simulink model "VCU_board_v8"  (R2019b)
settings: Solver=VariableStepAuto  StartTime=0.0  StopTime=300  RelTol=1e-3
undefined symbols (not defined in the file): canChannel
libraries: canmsglib x46, canlib x40
(part 1 of 2)
settings Model: EnablePacing=on  PacingRate=14  Creator=n10488456  LastModifiedBy=n10228748

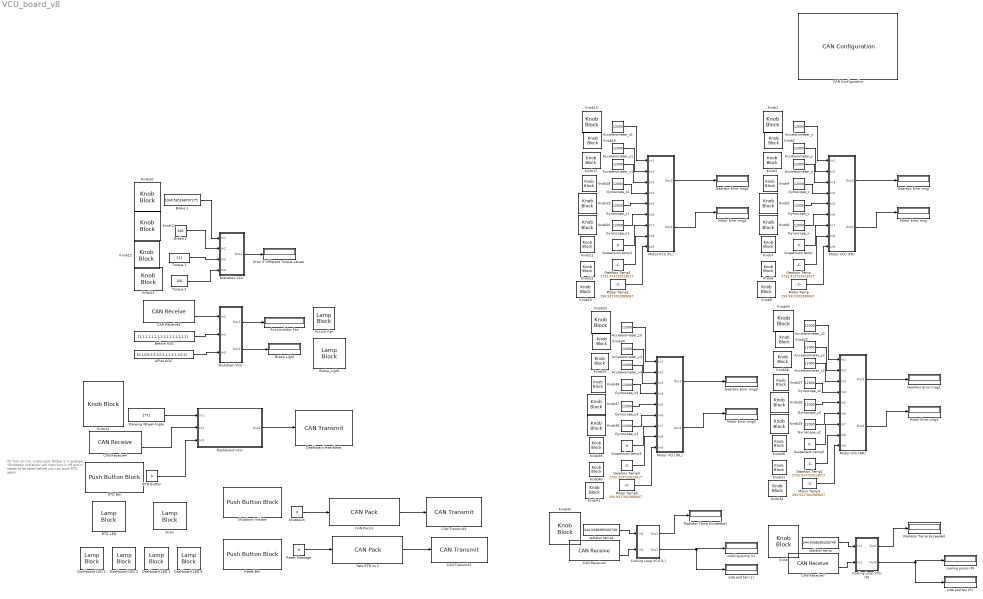
== system VCU_board_v8 ==
  note: To Turn on Car, make sure 'Brake 1' is pushed.
      | 'Shutdown initiation' will then turn it off and it needs to be reset before you can push RTD again.
  AFter ADC : Constant  Value=[0,1,0,0,1,0,1,0,1,1,1,1,1,1,0,1]
  Accelerometer_x{,1..3} (4 alike) : Constant  Value=12000  OutDataTypeStr=uint16
  Accelerometer_y{,1..3} (4 alike) : Constant  Value=12000  OutDataTypeStr=uint16
  Accelerometer_z{,1..3} (4 alike) : Constant  Value=12000  OutDataTypeStr=uint16
  Accum Fan : LampBlock
  Accumulator Fan : Display
  Before ADC : Constant  Value=[1,1,1,1,1,1,1,1,1,1,1,1,1,1,1,1]
  Brake 1 : Constant  Value=1040.565268707275
  Brake 2 : Constant  Value=100
  Brake Light : Display
  Brake_Light : LampBlock
  Brakebox VCU : Subsystem
  CAN Configuration : canlib/CAN Configuration  BlockHandle=69.0009  Device=MathWorks Virtual 1 (Channel 1)  DeviceMenu=MathWorks Virtual 1 (Channel 1)  ObjConstructor=canChannel('MathWorks', 'Virtual 1', 1)  BusSpeed=1000000  EnableBitParameters=off  AckMode=Normal
      settings: SourceProductName=Vehicle Network Toolbox  SourceProductBaseCode=VN
  CAN Pack3 : canmsglib/CAN Pack  MsgList=(none)  MsgName=Shutdown Notif  MsgIDType=Standard (11-bit identifier)  MsgIdentifier=62  MsgLength=1  Remote=off  ApplyMinMax=off  BusOutput=off  SignalInfo={ 'Signal1', '0', '1', 'LE', 'unsigned', 'Standard', '0', '1', '0', '-Inf', 'Inf' }
      settings: SourceProductName=Vehicle Network Toolbox  SourceProductBaseCode=VN  DataFormat=manually specified signals
  CAN Receive1 : canlib/CAN Receive  BlockHandle=71.0007  Device=MathWorks Virtual 1 (Channel 1)  DeviceMenu=MathWorks Virtual 1 (Channel 1)  ObjConstructor=canChannel('MathWorks', 'Virtual 1', 1)  EnableStandardIDsFilter=off  StdIDsCombo=Allow only  StandardIDs=[41 61]  EnableExtendedIDsFilter=off  ExtIDsCombo=Allow all  ExtendedIDs=0  SampleTime=0.01  MsgsPerTimestep=all  InternalFilterUpdateStatus=on  BusOutput=off
      settings: SourceProductName=Vehicle Network Toolbox  SourceProductBaseCode=VN
  CAN Receive4 : canlib/CAN Receive  BlockHandle=72.0004  Device=MathWorks Virtual 1 (Channel 1)  DeviceMenu=MathWorks Virtual 1 (Channel 1)  ObjConstructor=canChannel('MathWorks', 'Virtual 1', 1)  EnableStandardIDsFilter=off  StdIDsCombo=Allow only  StandardIDs=[22 51 61 62]  EnableExtendedIDsFilter=off  ExtIDsCombo=Allow all  ExtendedIDs=0  SampleTime=0.01  MsgsPerTimestep=all  InternalFilterUpdateStatus=on  BusOutput=off
      settings: SourceProductName=Vehicle Network Toolbox  SourceProductBaseCode=VN
  CAN Receive5 : canlib/CAN Receive  BlockHandle=73.0004  Device=MathWorks Virtual 1 (Channel 1)  DeviceMenu=MathWorks Virtual 1 (Channel 1)  ObjConstructor=canChannel('MathWorks', 'Virtual 1', 1)  EnableStandardIDsFilter=off  StdIDsCombo=Allow only  StandardIDs=[41 51 61]  EnableExtendedIDsFilter=off  ExtIDsCombo=Allow all  ExtendedIDs=0  SampleTime=0.01  MsgsPerTimestep=all  InternalFilterUpdateStatus=on  BusOutput=off
      settings: SourceProductName=Vehicle Network Toolbox  SourceProductBaseCode=VN
  CAN Receive7 : canlib/CAN Receive  BlockHandle=74.0004  Device=MathWorks Virtual 1 (Channel 1)  DeviceMenu=MathWorks Virtual 1 (Channel 1)  ObjConstructor=canChannel('MathWorks', 'Virtual 1', 1)  EnableStandardIDsFilter=off  StdIDsCombo=Allow only  StandardIDs=[41 61]  EnableExtendedIDsFilter=off  ExtIDsCombo=Allow all  ExtendedIDs=0  SampleTime=0.01  MsgsPerTimestep=all  InternalFilterUpdateStatus=on  BusOutput=off
      settings: SourceProductName=Vehicle Network Toolbox  SourceProductBaseCode=VN
  CAN Transmit1 : canlib/CAN Transmit  BlockHandle=76.0004  Device=MathWorks Virtual 1 (Channel 1)  DeviceMenu=MathWorks Virtual 1 (Channel 1)  ObjConstructor=canChannel('MathWorks', 'Virtual 1', 1)  EnablePeriodicTransmit=on  MessagePeriod=0.250
      settings: SourceProductName=Vehicle Network Toolbox  SourceProductBaseCode=VN
  CAN Transmit3 : canlib/CAN Transmit  BlockHandle=77.0004  Device=MathWorks Virtual 1 (Channel 1)  DeviceMenu=MathWorks Virtual 1 (Channel 1)  ObjConstructor=canChannel('MathWorks', 'Virtual 1', 1)  EnablePeriodicTransmit=on  MessagePeriod=0.250
      settings: SourceProductName=Vehicle Network Toolbox  SourceProductBaseCode=VN
  Cooling Loop VCU (L) : Subsystem
  Cooling Loop VCU (R) : Subsystem
  Dashboard Heartbeat : canlib/CAN Transmit  BlockHandle=209.0004  Device=MathWorks Virtual 1 (Channel 1)  DeviceMenu=MathWorks Virtual 1 (Channel 1)  ObjConstructor=canChannel('MathWorks', 'Virtual 1', 1)  EnablePeriodicTransmit=on  MessagePeriod=0.250
      settings: SourceProductName=Vehicle Network Toolbox  SourceProductBaseCode=VN
  Dashboard LED {1..4} (4 alike) : LampBlock
  Dashboard VCU : Subsystem
  Error if different Torque values : Display
  Gearbox Error msg{,1..3} (4 alike) : Display
  Gearbox Temp{,1..3} (4 alike) : Constant  Value=2732.414722614017  OutDataTypeStr=uint16
  Gyroscope_x{,1..3} (4 alike) : Constant  Value=12000  OutDataTypeStr=uint16
  Gyroscope_y{,1..3} (4 alike) : Constant  Value=12000  OutDataTypeStr=uint16
  Gyroscope_z{,1..3} (4 alike) : Constant  Value=12000  OutDataTypeStr=uint16
  Knob{,7..14,21..23,30..32,39..42} (19 alike) : KnobBlock  ScaleMax=4095
  Knob{1..6,15..20,24..29,33..38} (24 alike) : KnobBlock  ScaleMax=65535
  Motor Error msg{,1..3} (4 alike) : Display
  Motor Temp{,1..3} (4 alike) : Constant  Value=294.9317002989067  OutDataTypeStr=uint16
  Motor VCU (FL) : Subsystem
  Motor VCU (FR) : Subsystem
  Motor VCU (RL) : Subsystem
  Motor VCU (RR) : Subsystem
  RTD Btn : PushButtonBlock  ButtonText=RTD Button
  RTD Button : Constant  Value=0  OutDataTypeStr=boolean  SampleTime=0.1
  RTD LED : LampBlock
  Radiator Temp Exceeded : Display
  Radiator Temp Exceeded1 : Display
  Reset Btn : PushButtonBlock  ButtonText=Reset Button
  Reset Message : Constant  Value=0
  Sets RTD to 2 : canmsglib/CAN Pack  MsgList=(none)  MsgName=RTD Notif  MsgIDType=Standard (11-bit identifier)  MsgIdentifier=61  MsgLength=1  Remote=off  ApplyMinMax=off  BusOutput=off  SignalInfo={ 'Signal1', '0', '1', 'LE', 'unsigned', 'Standard', '0', '1', '0', '-Inf', 'Inf' }
      settings: SourceProductName=Vehicle Network Toolbox  SourceProductBaseCode=VN  DataFormat=manually specified signals
  Shutdown : Constant  Value=0
  Shutdown Initiate : PushButtonBlock  ButtonText=Shutdown Initiate
  Shutdown VCU : Subsystem
  Siren : LampBlock
  Stereing Wheel Angle : Constant  Value=1771  OutDataTypeStr=uint16  SampleTime=0.1
  Suspension temp{,1..3} (4 alike) : Constant  Value=0  OutDataTypeStr=uint16
  Torque 1 : Constant  Value=111
  Torque 2 : Constant  Value=100
  cooling pump (L) : Display
  cooling pump (R) : Display
  radiator temp : Constant  Value=244.5438395200749  OutDataTypeStr=uint16
  radiator temp1 : Constant  Value=244.5438395200749  OutDataTypeStr=uint16
  side pod fan (L) : Display
  side pod fan (R) : Display
  wires:
  Accelerometer_z/1 -> Motor VCU (FR)/1(In1)
  Accelerometer_y/1 -> Motor VCU (FR)/2(In2)
  Accelerometer_x/1 -> Motor VCU (FR)/3(In3)
  Gyroscope_z/1 -> Motor VCU (FR)/4(In4)
  Gyroscope_y/1 -> Motor VCU (FR)/5(In5)
  Gyroscope_x/1 -> Motor VCU (FR)/6(In6)
  Suspension temp/1 -> Motor VCU (FR)/7(In7)
  Gearbox Temp/1 -> Motor VCU (FR)/8(In8)
  Motor Temp/1 -> Motor VCU (FR)/9(In9)
  Motor VCU (FR)/1(Out3) -> Gearbox Error msg/1
  Motor VCU (FR)/2(Out4) -> Motor Error msg/1
  Brakebox VCU/1(Out2) -> Error if different Torque values/1
  Brake 2/1 -> Brakebox VCU/2(In2)
  Brake 1/1 -> Brakebox VCU/1(In1)
  Torque 2/1 -> Brakebox VCU/4(In4)
  Torque 1/1 -> Brakebox VCU/3(In3)
  CAN Receive4/2 -> Dashboard VCU/2(In2)
  Stereing Wheel Angle/1 -> Dashboard VCU/1(In1)
  Dashboard VCU/1(Out1) -> Dashboard Heartbeat/1
  RTD Button/1 -> Dashboard VCU/3(In3)
  Cooling Loop VCU (R)/2(Out3) -> side pod fan (R)/1, cooling pump (R)/1
  radiator temp/1 -> Cooling Loop VCU (R)/1(In1)
  CAN Receive7/2 -> Cooling Loop VCU (R)/2(In2)
  Cooling Loop VCU (R)/1(Out1) -> Radiator Temp Exceeded/1
  CAN Receive5/2 -> Shutdown VCU/1(In2)
  Shutdown VCU/2(Out2) -> Brake Light/1
  AFter ADC/1 -> Shutdown VCU/3(In5)
  Shutdown VCU/1(Out1) -> Accumulator Fan/1
  Before ADC/1 -> Shutdown VCU/2(In3)
  Shutdown/1 -> CAN Pack3/1
  CAN Pack3/1 -> CAN Transmit3/1
  Reset Message/1 -> Sets RTD to 2/1
  Sets RTD to 2/1 -> CAN Transmit1/1
  Accelerometer_y1/1 -> Motor VCU (FL)/2(In2)
  Motor Temp1/1 -> Motor VCU (FL)/9(In9)
  Gearbox Temp1/1 -> Motor VCU (FL)/8(In8)
  Gyroscope_z1/1 -> Motor VCU (FL)/4(In4)
  Motor VCU (FL)/1(Out3) -> Gearbox Error msg1/1
  Suspension temp1/1 -> Motor VCU (FL)/7(In7)
  Accelerometer_z1/1 -> Motor VCU (FL)/1(In1)
  Accelerometer_x1/1 -> Motor VCU (FL)/3(In3)
  Motor VCU (FL)/2(Out4) -> Motor Error msg1/1
  Gyroscope_x1/1 -> Motor VCU (FL)/6(In6)
  Gyroscope_y1/1 -> Motor VCU (FL)/5(In5)
  Accelerometer_y2/1 -> Motor VCU (RR)/2(In2)
  Motor Temp2/1 -> Motor VCU (RR)/9(In9)
  Gearbox Temp2/1 -> Motor VCU (RR)/8(In8)
  Gyroscope_z2/1 -> Motor VCU (RR)/4(In4)
  Motor VCU (RR)/1(Out3) -> Gearbox Error msg2/1
  Suspension temp2/1 -> Motor VCU (RR)/7(In7)
  Accelerometer_z2/1 -> Motor VCU (RR)/1(In1)
  Accelerometer_x2/1 -> Motor VCU (RR)/3(In3)
  Motor VCU (RR)/2(Out4) -> Motor Error msg2/1
  Gyroscope_x2/1 -> Motor VCU (RR)/6(In6)
  Gyroscope_y2/1 -> Motor VCU (RR)/5(In5)
  Accelerometer_y3/1 -> Motor VCU (RL)/2(In2)
  Motor Temp3/1 -> Motor VCU (RL)/9(In9)
  Gearbox Temp3/1 -> Motor VCU (RL)/8(In8)
  Gyroscope_z3/1 -> Motor VCU (RL)/4(In4)
  Motor VCU (RL)/1(Out3) -> Gearbox Error msg3/1
  Suspension temp3/1 -> Motor VCU (RL)/7(In7)
  Accelerometer_z3/1 -> Motor VCU (RL)/1(In1)
  Accelerometer_x3/1 -> Motor VCU (RL)/3(In3)
  Motor VCU (RL)/2(Out4) -> Motor Error msg3/1
  Gyroscope_x3/1 -> Motor VCU (RL)/6(In6)
  Gyroscope_y3/1 -> Motor VCU (RL)/5(In5)
  Cooling Loop VCU (L)/1(Out1) -> Radiator Temp Exceeded1/1
  radiator temp1/1 -> Cooling Loop VCU (L)/1(In1)
  Cooling Loop VCU (L)/2(Out3) -> side pod fan (L)/1, cooling pump (L)/1
  CAN Receive1/2 -> Cooling Loop VCU (L)/2(In2)

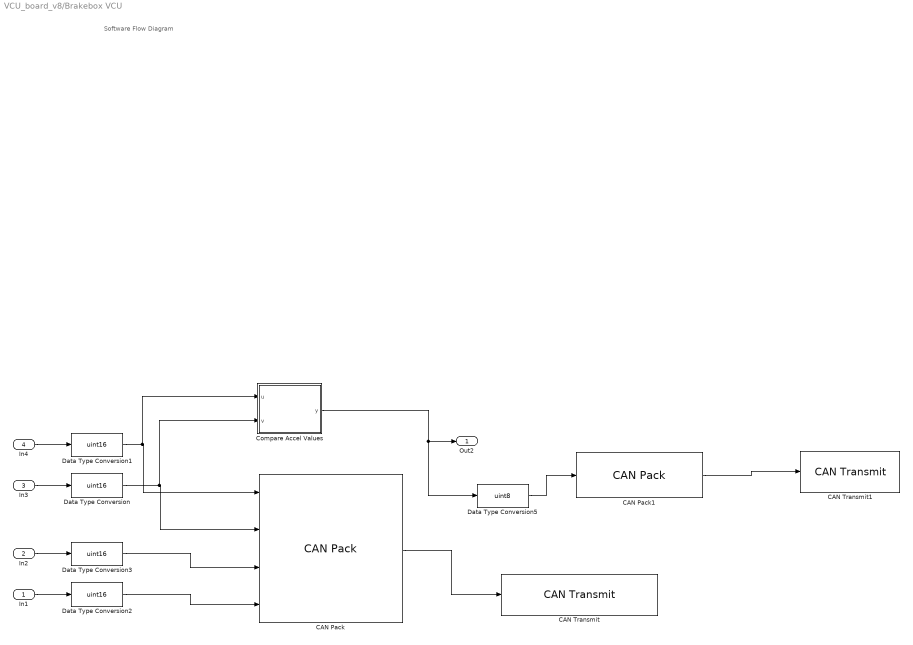
== system VCU_board_v8/Brakebox VCU ==
  note: Software Flow Diagram
  In1 : Inport
  In2 : Inport  Port=2
  In3 : Inport  Port=3
  In4 : Inport  Port=4
  CAN Pack : canmsglib/CAN Pack  MsgList=(none)  MsgName=CAN Msg  MsgIDType=Standard (11-bit identifier)  MsgIdentifier=51  MsgLength=6  Remote=off  ApplyMinMax=off  BusOutput=off  SignalInfo={ 'Torque2', '0', '12', 'LE', 'unsigned', 'Standard', '0', '1', '0', '-Inf', 'Inf'; 'Torque1', '12', '12', 'LE', 'unsigned', 'Standard', '0', '1', '0', '-Inf', 'Inf'; 'BrakePos', '24', '12', 'LE', 'unsigned', 'Standard', '0', '1', '0', '-Inf', 'Inf'; 'BrakePres', '36', '12', 'LE', 'unsigned', 'Standard', '0', '1', '0', '-Inf', 'Inf' }
      settings: SourceProductName=Vehicle Network Toolbox  SourceProductBaseCode=VN  DataFormat=manually specified signals
  CAN Pack1 : canmsglib/CAN Pack  MsgList=(none)  MsgName=CAN Msg  MsgIDType=Standard (11-bit identifier)  MsgIdentifier=52  MsgLength=8  Remote=off  ApplyMinMax=off  BusOutput=off  SignalInfo="{  }"
      settings: SourceProductName=Vehicle Network Toolbox  SourceProductBaseCode=VN  DataFormat=raw data
  CAN Transmit : canlib/CAN Transmit  BlockHandle=19.0002  Device=MathWorks Virtual 1 (Channel 1)  DeviceMenu=MathWorks Virtual 1 (Channel 1)  ObjConstructor=canChannel('MathWorks', 'Virtual 1', 1)  EnablePeriodicTransmit=on  MessagePeriod=0.250
      settings: SourceProductName=Vehicle Network Toolbox  SourceProductBaseCode=VN
  CAN Transmit1 : canlib/CAN Transmit  BlockHandle=20.0002  Device=MathWorks Virtual 1 (Channel 1)  DeviceMenu=MathWorks Virtual 1 (Channel 1)  ObjConstructor=canChannel('MathWorks', 'Virtual 1', 1)  EnablePeriodicTransmit=on  MessagePeriod=0.250
      settings: SourceProductName=Vehicle Network Toolbox  SourceProductBaseCode=VN
  Compare Accel Values : MATLAB Function  TreatAsAtomicUnit=on
  Data Type Conversion{,1..3} (4 alike) : DataTypeConversion  OutDataTypeStr=uint16
  Data Type Conversion5 : DataTypeConversion  OutDataTypeStr=uint8
  Out2 : Outport
  wires:
  In2/1 -> Data Type Conversion3/1
  Data Type Conversion/1 -> Compare Accel Values/2(v), CAN Pack/2
  Data Type Conversion1/1 -> Compare Accel Values/1(u), CAN Pack/1
  In3/1 -> Data Type Conversion/1
  In1/1 -> Data Type Conversion2/1
  Compare Accel Values/1(y) -> Data Type Conversion5/1, Out2/1
  In4/1 -> Data Type Conversion1/1
  CAN Pack/1 -> CAN Transmit/1
  CAN Pack1/1 -> CAN Transmit1/1
  Data Type Conversion5/1 -> CAN Pack1/1
  Data Type Conversion2/1 -> CAN Pack/4
  Data Type Conversion3/1 -> CAN Pack/3

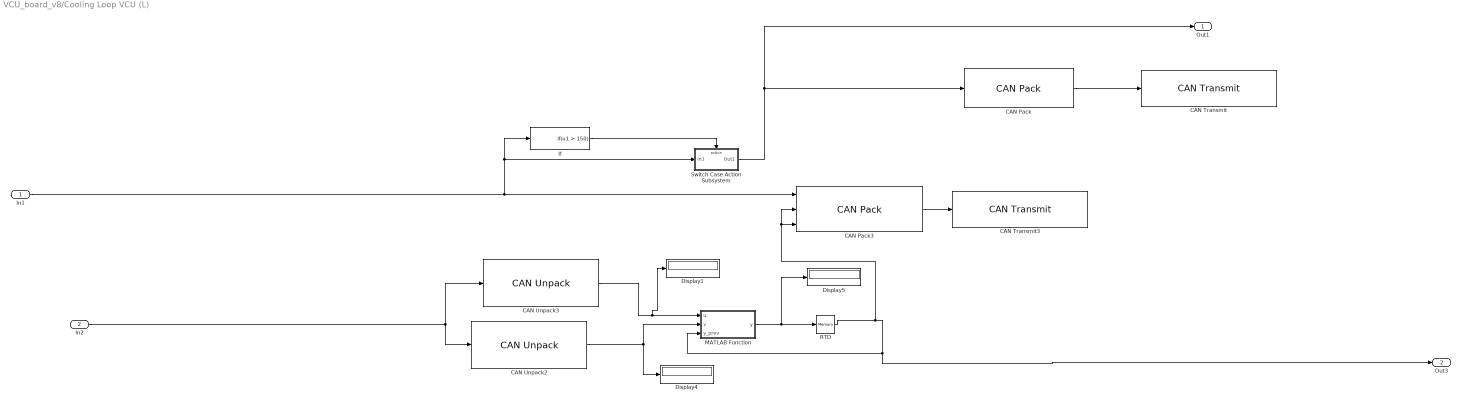
== system VCU_board_v8/Cooling Loop VCU (L) ==
  In1 : Inport
  In2 : Inport  Port=2
  CAN Pack : canmsglib/CAN Pack  MsgList=(none)  MsgName=Error RadiatorT L  MsgIDType=Standard (11-bit identifier)  MsgIdentifier=322  MsgLength=1  Remote=off  ApplyMinMax=off  BusOutput=off  SignalInfo={ 'Signal1', '0', '1', 'LE', 'unsigned', 'Standard', '0', '1', '0', '-Inf', 'Inf' }
      settings: SourceProductName=Vehicle Network Toolbox  SourceProductBaseCode=VN  DataFormat=manually specified signals
  CAN Pack3 : canmsglib/CAN Pack  MsgList=(none)  MsgName=Cooling Loop Heartbeat L  MsgIDType=Standard (11-bit identifier)  MsgIdentifier=312  MsgLength=2  Remote=off  ApplyMinMax=off  BusOutput=off  SignalInfo={ 'RadiatorT', '0', '12', 'LE', 'unsigned', 'Standard', '0', '1', '0', '-Inf', 'Inf'; 'SideFan', '12', '1', 'LE', 'unsigned', 'Standard', '0', '1', '0', '-Inf', 'Inf'; 'Pump', '13', '1', 'LE', 'unsigned', 'Standard', '0', '1', '0', '-Inf', 'Inf' }
      settings: SourceProductName=Vehicle Network Toolbox  SourceProductBaseCode=VN  DataFormat=manually specified signals
  CAN Transmit : canlib/CAN Transmit  BlockHandle=78.0002  Device=MathWorks Virtual 1 (Channel 1)  DeviceMenu=MathWorks Virtual 1 (Channel 1)  ObjConstructor=canChannel('MathWorks', 'Virtual 1', 1)  EnablePeriodicTransmit=on  MessagePeriod=0.250
      settings: SourceProductName=Vehicle Network Toolbox  SourceProductBaseCode=VN
  CAN Transmit3 : canlib/CAN Transmit  BlockHandle=79.0002  Device=MathWorks Virtual 1 (Channel 1)  DeviceMenu=MathWorks Virtual 1 (Channel 1)  ObjConstructor=canChannel('MathWorks', 'Virtual 1', 1)  EnablePeriodicTransmit=on  MessagePeriod=0.250
      settings: SourceProductName=Vehicle Network Toolbox  SourceProductBaseCode=VN
  CAN Unpack2 : canmsglib/CAN Unpack  MsgList=(none)  MsgName=Reset Notif  MsgIDType=Standard (11-bit identifier)  MsgIdentifier=61  MsgLength=1  SignalInfo={ 'Reset', '0', '1', 'LE', 'unsigned', 'Standard', '0', '1', '0', '-Inf', 'Inf' }  IDPort=off  TimestampPort=off  ErrorPort=off  RemotePort=off  LengthPort=off  StatusPort=off  ApplyMinMax=off
      settings: SourceProductName=Vehicle Network Toolbox  SourceProductBaseCode=VN
  CAN Unpack3 : canmsglib/CAN Unpack  MsgList=(none)  MsgName=RTD Notif  MsgIDType=Standard (11-bit identifier)  MsgIdentifier=41  MsgLength=3  SignalInfo={ 'RTD', '0', '1', 'LE', 'unsigned', 'Standard', '0', '1', '0', '-Inf', 'Inf' }  IDPort=off  TimestampPort=off  ErrorPort=off  RemotePort=off  LengthPort=off  StatusPort=off  ApplyMinMax=off
      settings: SourceProductName=Vehicle Network Toolbox  SourceProductBaseCode=VN
  Display1 : Display
  Display4 : Display
  Display5 : Display
  If : If  IfExpression=u1 > 150  ShowElse=off
  MATLAB Function : MATLAB Function  TreatAsAtomicUnit=on
  RTD : Memory  InheritSampleTime=on
  Switch Case Action Subsystem : Subsystem  TreatAsAtomicUnit=on
  Out1 : Outport
  Out3 : Outport  Port=2
  wires:
  In1/1 -> CAN Pack3/1, If/1, Switch Case Action Subsystem/1(In1)
  Switch Case Action Subsystem/1(Out1) -> CAN Pack/1, Out1/1
  CAN Pack/1 -> CAN Transmit/1
  CAN Pack3/1 -> CAN Transmit3/1
  If/1 -> Switch Case Action Subsystem/Action
  CAN Unpack2/1 -> Display4/1, MATLAB Function/2(v)
  CAN Unpack3/1 -> Display1/1, MATLAB Function/1(u)
  In2/1 -> CAN Unpack3/1, CAN Unpack2/1
  MATLAB Function/1(y) -> Display5/1, RTD/1
  RTD/1 -> Out3/1, MATLAB Function/3(y_prev), CAN Pack3/3, CAN Pack3/2

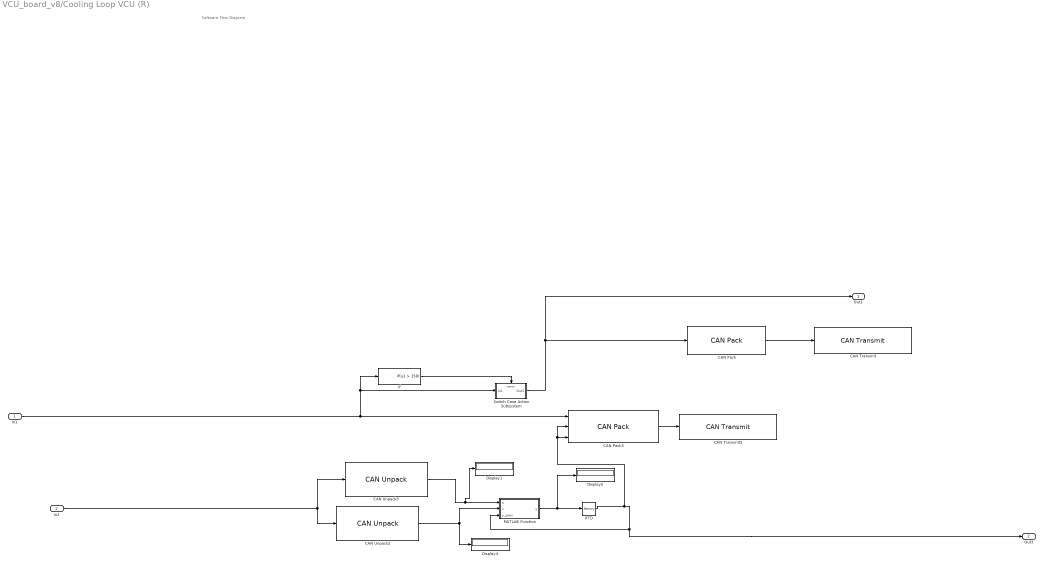
== system VCU_board_v8/Cooling Loop VCU (R) ==
  note: Software Flow Diagram
  In1 : Inport
  In2 : Inport  Port=2
  CAN Pack : canmsglib/CAN Pack  MsgList=(none)  MsgName=Error RadiatorT  MsgIDType=Standard (11-bit identifier)  MsgIdentifier=321  MsgLength=1  Remote=off  ApplyMinMax=off  BusOutput=off  SignalInfo={ 'Signal1', '0', '1', 'LE', 'unsigned', 'Standard', '0', '1', '0', '-Inf', 'Inf' }
      settings: SourceProductName=Vehicle Network Toolbox  SourceProductBaseCode=VN  DataFormat=manually specified signals
  CAN Pack3 : canmsglib/CAN Pack  MsgList=(none)  MsgName=Cooling Loop Heartbeat  MsgIDType=Standard (11-bit identifier)  MsgIdentifier=311  MsgLength=2  Remote=off  ApplyMinMax=off  BusOutput=off  SignalInfo={ 'RadiatorT', '0', '12', 'LE', 'unsigned', 'Standard', '0', '1', '0', '-Inf', 'Inf'; 'SideFan', '12', '1', 'LE', 'unsigned', 'Standard', '0', '1', '0', '-Inf', 'Inf'; 'Pump', '13', '1', 'LE', 'unsigned', 'Standard', '0', '1', '0', '-Inf', 'Inf' }
      settings: SourceProductName=Vehicle Network Toolbox  SourceProductBaseCode=VN  DataFormat=manually specified signals
  CAN Transmit : canlib/CAN Transmit  BlockHandle=78.0002  Device=MathWorks Virtual 1 (Channel 1)  DeviceMenu=MathWorks Virtual 1 (Channel 1)  ObjConstructor=canChannel('MathWorks', 'Virtual 1', 1)  EnablePeriodicTransmit=on  MessagePeriod=0.250
      settings: SourceProductName=Vehicle Network Toolbox  SourceProductBaseCode=VN
  CAN Transmit3 : canlib/CAN Transmit  BlockHandle=79.0002  Device=MathWorks Virtual 1 (Channel 1)  DeviceMenu=MathWorks Virtual 1 (Channel 1)  ObjConstructor=canChannel('MathWorks', 'Virtual 1', 1)  EnablePeriodicTransmit=on  MessagePeriod=0.250
      settings: SourceProductName=Vehicle Network Toolbox  SourceProductBaseCode=VN
  CAN Unpack2 : canmsglib/CAN Unpack  MsgList=(none)  MsgName=Reset Notif  MsgIDType=Standard (11-bit identifier)  MsgIdentifier=61  MsgLength=1  SignalInfo={ 'Reset', '0', '1', 'LE', 'unsigned', 'Standard', '0', '1', '0', '-Inf', 'Inf' }  IDPort=off  TimestampPort=off  ErrorPort=off  RemotePort=off  LengthPort=off  StatusPort=off  ApplyMinMax=off
      settings: SourceProductName=Vehicle Network Toolbox  SourceProductBaseCode=VN
  CAN Unpack3 : canmsglib/CAN Unpack  MsgList=(none)  MsgName=RTD Notif  MsgIDType=Standard (11-bit identifier)  MsgIdentifier=41  MsgLength=3  SignalInfo={ 'RTD', '0', '1', 'LE', 'unsigned', 'Standard', '0', '1', '0', '-Inf', 'Inf' }  IDPort=off  TimestampPort=off  ErrorPort=off  RemotePort=off  LengthPort=off  StatusPort=off  ApplyMinMax=off
      settings: SourceProductName=Vehicle Network Toolbox  SourceProductBaseCode=VN
  Display1 : Display
  Display4 : Display
  Display5 : Display
  If : If  IfExpression=u1 > 150  ShowElse=off
  MATLAB Function : MATLAB Function  TreatAsAtomicUnit=on
  RTD : Memory  InheritSampleTime=on
  Switch Case Action Subsystem : Subsystem  TreatAsAtomicUnit=on
  Out1 : Outport
  Out3 : Outport  Port=2
  wires:
  In1/1 -> CAN Pack3/1, If/1, Switch Case Action Subsystem/1(In1)
  Switch Case Action Subsystem/1(Out1) -> CAN Pack/1, Out1/1
  CAN Pack/1 -> CAN Transmit/1
  CAN Pack3/1 -> CAN Transmit3/1
  If/1 -> Switch Case Action Subsystem/Action
  CAN Unpack2/1 -> Display4/1, MATLAB Function/2(v)
  CAN Unpack3/1 -> Display1/1, MATLAB Function/1(u)
  In2/1 -> CAN Unpack3/1, CAN Unpack2/1
  MATLAB Function/1(y) -> Display5/1, RTD/1
  RTD/1 -> Out3/1, MATLAB Function/3(y_prev), CAN Pack3/3, CAN Pack3/2

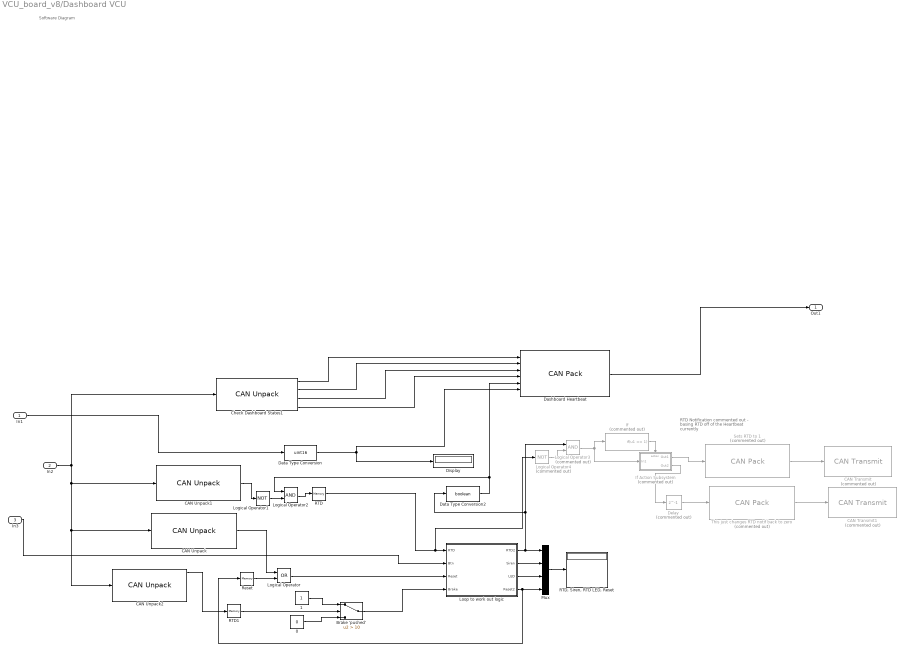
== system VCU_board_v8/Dashboard VCU ==
  note: Software Diagram
  note: RTD Notification commented out - basing RTD off of the Heartbeat currently
  In1 : Inport
  In2 : Inport  Port=2
  In3 : Inport  Port=3
  0 : Constant  Value=0  OutDataTypeStr=boolean
  1 : Constant  OutDataTypeStr=boolean  SampleTime=0.1
  Brake 'pushed' : Switch  Criteria=u2 > Threshold  Threshold=10
  CAN Transmit : canlib/CAN Transmit  Commented=on  BlockHandle=221.0007  Device=MathWorks Virtual 1 (Channel 1)  DeviceMenu=MathWorks Virtual 1 (Channel 1)  ObjConstructor=canChannel('MathWorks', 'Virtual 1', 1)  EnablePeriodicTransmit=off  MessagePeriod=1.000
      settings: SourceProductName=Vehicle Network Toolbox  SourceProductBaseCode=VN
  CAN Transmit1 : canlib/CAN Transmit  Commented=on  BlockHandle=222.0004  Device=MathWorks Virtual 1 (Channel 1)  DeviceMenu=MathWorks Virtual 1 (Channel 1)  ObjConstructor=canChannel('MathWorks', 'Virtual 1', 1)  EnablePeriodicTransmit=off  MessagePeriod=1.000
      settings: SourceProductName=Vehicle Network Toolbox  SourceProductBaseCode=VN
  CAN Unpack : canmsglib/CAN Unpack  MsgList=(none)  MsgName=Reset Notif  MsgIDType=Standard (11-bit identifier)  MsgIdentifier=61  MsgLength=1  SignalInfo={ 'Reset', '0', '1', 'LE', 'unsigned', 'Standard', '0', '1', '0', '-Inf', 'Inf' }  IDPort=off  TimestampPort=off  ErrorPort=off  RemotePort=off  LengthPort=off  StatusPort=off  ApplyMinMax=off
      settings: SourceProductName=Vehicle Network Toolbox  SourceProductBaseCode=VN
  CAN Unpack1 : canmsglib/CAN Unpack  MsgList=(none)  MsgName=Shutdown Notif  MsgIDType=Standard (11-bit identifier)  MsgIdentifier=62  MsgLength=1  SignalInfo={ 'Shtdwn', '0', '1', 'LE', 'unsigned', 'Standard', '0', '1', '0', '-Inf', 'Inf' }  IDPort=off  TimestampPort=off  ErrorPort=off  RemotePort=off  LengthPort=off  StatusPort=off  ApplyMinMax=off
      settings: SourceProductName=Vehicle Network Toolbox  SourceProductBaseCode=VN
  CAN Unpack2 : canmsglib/CAN Unpack  MsgList=(none)  MsgName=CAN Msg  MsgIDType=Standard (11-bit identifier)  MsgIdentifier=51  MsgLength=6  SignalInfo={ 'BrakePres', '36', '12', 'LE', 'unsigned', 'Standard', '0', '1', '0', '-Inf', 'Inf'; 'Brake2', '24', '12', 'LE', 'unsigned', 'Standard', '0', '1', '0', '-Inf', 'Inf'; 'Torque1', '12', '12', 'LE', 'unsigned', 'Standard', '0', '1', '0', '-Inf', 'Inf'; 'Torque2', '0', '12', 'LE', 'unsigned', 'Standard', '0', '1', '0', '-Inf', 'Inf' }  IDPort=off  TimestampPort=off  ErrorPort=off  RemotePort=off  LengthPort=off  StatusPort=off  ApplyMinMax=off
      settings: SourceProductName=Vehicle Network Toolbox  SourceProductBaseCode=VN
  Check Dashboard States1 : canmsglib/CAN Unpack  MsgList=(none)  MsgName=CAN Msg  MsgIDType=Standard (11-bit identifier)  MsgIdentifier=22  MsgLength=3  SignalInfo={ 'Shutdown1', '8', '1', 'LE', 'unsigned', 'Standard', '0', '1', '0', '-Inf', 'Inf'; 'Shutdown2', '9', '1', 'LE', 'unsigned', 'Standard', '0', '1', '0', '-Inf', 'Inf'; 'Shutdown3', '10', '1', 'LE', 'unsigned', 'Standard', '0', '1', '0', '-Inf', 'Inf'; 'Shutdown4', '11', '1', 'LE', 'unsigned', 'Standard', '0', '1', '0', '-Inf', 'Inf' }  IDPort=off  TimestampPort=off  ErrorPort=off  RemotePort=off  LengthPort=off  StatusPort=off  ApplyMinMax=off
      settings: SourceProductName=Vehicle Network Toolbox  SourceProductBaseCode=VN
  Dashboard Heartbeat : canmsglib/CAN Pack  MsgList=(none)  MsgName=Dash Heartbeat  MsgIDType=Standard (11-bit identifier)  MsgIdentifier=41  MsgLength=3  Remote=off  ApplyMinMax=off  BusOutput=off  SignalInfo={ 'Dash1', '20', '1', 'LE', 'unsigned', 'Standard', '0', '1', '0', '-Inf', 'Inf'; 'Dash2', '21', '1', 'LE', 'unsigned', 'Standard', '0', '1', '0', '-Inf', 'Inf'; 'Dash3', '22', '1', 'LE', 'unsigned', 'Standard', '0', '1', '0', '-Inf', 'Inf'; 'Dash4', '23', '1', 'LE', 'unsigned', 'Standard', '0', '1', '0', '-Inf', 'Inf'; 'RTD State', '0', '1', 'LE', 'unsigned', 'Standard', '0', '1', '0', '-Inf', 'Inf'; 'SteeringWheel', '8', '12', 'LE', 'unsigned', 'Standard', '0', '1', '0', '-Inf', 'Inf' }
      settings: SourceProductName=Vehicle Network Toolbox  SourceProductBaseCode=VN  DataFormat=manually specified signals
  Data Type Conversion : DataTypeConversion  OutDataTypeStr=uint16
  Data Type Conversion2 : DataTypeConversion  OutDataTypeStr=boolean
  Delay : Delay  Commented=on  DelayLength=1  InitialCondition=0
  Display : Display
  If : If  Commented=on  IfExpression=u1 == 1  ShowElse=off
  If Action Subsystem : Subsystem  Commented=on  TreatAsAtomicUnit=on
  Logical Operator : Logic  Operator=OR  AllPortsSameDT=off  OutDataTypeStr=boolean
  Logical Operator1 : Logic  Operator=NOT  AllPortsSameDT=off  OutDataTypeStr=boolean
  Logical Operator2 : Logic  AllPortsSameDT=off  OutDataTypeStr=boolean
  Logical Operator3 : Logic  Commented=on  AllPortsSameDT=off  OutDataTypeStr=boolean
  Logical Operator4 : Logic  Commented=on  Operator=NOT  AllPortsSameDT=off  OutDataTypeStr=boolean
  Loop to work out logic : MATLAB Function  TreatAsAtomicUnit=on
  Mux : Mux
  RTD : Memory  InheritSampleTime=on
  "RTD, Siren, RTD LED, Reset" : Display
  RTD1 : Memory  InheritSampleTime=on
  Reset : Memory  InitialCondition=1  InheritSampleTime=on
  Sets RTD to 1 : canmsglib/CAN Pack  Commented=on  MsgList=(none)  MsgName=RTD Notif  MsgIDType=Standard (11-bit identifier)  MsgIdentifier=42  MsgLength=1  Remote=off  ApplyMinMax=off  BusOutput=off  SignalInfo={ 'Signal1', '0', '1', 'LE', 'unsigned', 'Standard', '0', '1', '0', '-Inf', 'Inf' }
      settings: SourceProductName=Vehicle Network Toolbox  SourceProductBaseCode=VN  DataFormat=manually specified signals
  This just changes RTD notif back to zero : canmsglib/CAN Pack  Commented=on  MsgList=(none)  MsgName=RTD Notif  MsgIDType=Standard (11-bit identifier)  MsgIdentifier=42  MsgLength=1  Remote=off  ApplyMinMax=off  BusOutput=off  SignalInfo={ 'Signal1', '0', '1', 'LE', 'unsigned', 'Standard', '0', '1', '0', '-Inf', 'Inf' }
      settings: SourceProductName=Vehicle Network Toolbox  SourceProductBaseCode=VN  DataFormat=manually specified signals
  Out1 : Outport
  wires:
  Mux/1 -> "RTD, Siren, RTD LED, Reset"/1
  Data Type Conversion2/1 -> Dashboard Heartbeat/5, Logical Operator2/1
  Check Dashboard States1/4 -> Dashboard Heartbeat/4
  CAN Unpack2/1 -> RTD1/1
  RTD1/1 -> Brake 'pushed'/2
  Dashboard Heartbeat/1 -> Out1/1
  Brake 'pushed'/1 -> Loop to work out logic/4(Brake)
  Check Dashboard States1/2 -> Dashboard Heartbeat/2
  Logical Operator/1 -> Loop to work out logic/3(Reset)
  Check Dashboard States1/3 -> Dashboard Heartbeat/3
  RTD/1 -> Logical Operator4/1, Loop to work out logic/1(RTD)
  Loop to work out logic/3(LED) -> Mux/3
  0/1 -> Brake 'pushed'/3
  Loop to work out logic/2(Siren) -> Mux/2
  1/1 -> Brake 'pushed'/1
  Loop to work out logic/1(RTD2) -> Data Type Conversion2/1, Logical Operator3/1, Mux/1
  In2/1 -> CAN Unpack2/1, CAN Unpack/1, CAN Unpack1/1, Check Dashboard States1/1
  Check Dashboard States1/1 -> Dashboard Heartbeat/1
  In3/1 -> Loop to work out logic/2(Btn)
  Data Type Conversion/1 -> Dashboard Heartbeat/6, Display/1
  Loop to work out logic/4(Reset2) -> Reset/1, Mux/4
  CAN Unpack/1 -> Logical Operator/1
  Reset/1 -> Logical Operator/2
  In1/1 -> Data Type Conversion/1
  Logical Operator2/1 -> RTD/1
  CAN Unpack1/1 -> Logical Operator1/1
  Logical Operator1/1 -> Logical Operator2/2
  Logical Operator3/1 -> If Action Subsystem/1(In1), If/1
  If/1 -> If Action Subsystem/Action
  Sets RTD to 1/1 -> CAN Transmit/1
  Logical Operator4/1 -> Logical Operator3/2
  If Action Subsystem/2(Out2) -> Delay/1
  If Action Subsystem/1(Out1) -> Sets RTD to 1/1
  This just changes RTD notif back to zero/1 -> CAN Transmit1/1
  Delay/1 -> This just changes RTD notif back to zero/1

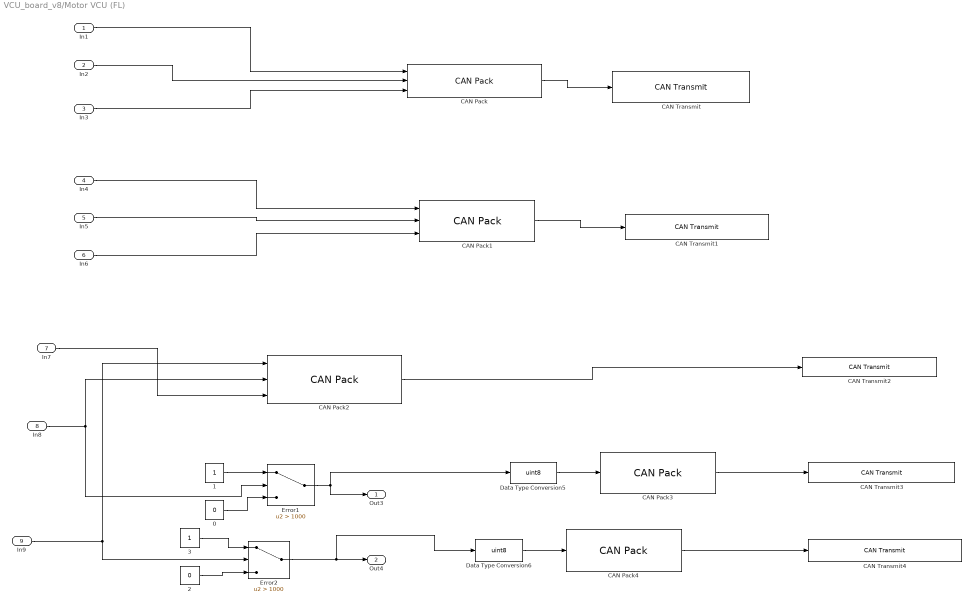
== system VCU_board_v8/Motor VCU (FL) ==
  In1 : Inport
  In2 : Inport  Port=2
  In3 : Inport  Port=3
  In4 : Inport  Port=4
  In5 : Inport  Port=5
  In6 : Inport  Port=6
  In7 : Inport  Port=7
  In8 : Inport  Port=8
  In9 : Inport  Port=9
  0 : Constant  Value=0
  1 : Constant
  2 : Constant  Value=0
  3 : Constant
  CAN Pack : canmsglib/CAN Pack  MsgList=(none)  MsgName=Accel FL  MsgIDType=Standard (11-bit identifier)  MsgIdentifier=153  MsgLength=6  Remote=off  ApplyMinMax=off  BusOutput=off  SignalInfo={ 'Accel_z', '0', '16', 'LE', 'unsigned', 'Standard', '0', '1', '0', '-Inf', 'Inf'; 'Accel_y', '16', '16', 'LE', 'unsigned', 'Standard', '0', '1', '0', '-Inf', 'Inf'; 'Accel_x', '32', '16', 'LE', 'unsigned', 'Standard', '0', '1', '0', '-Inf', 'Inf' }
      settings: SourceProductName=Vehicle Network Toolbox  SourceProductBaseCode=VN  DataFormat=manually specified signals
  CAN Pack1 : canmsglib/CAN Pack  MsgList=(none)  MsgName=Gyro FL  MsgIDType=Standard (11-bit identifier)  MsgIdentifier=143  MsgLength=6  Remote=off  ApplyMinMax=off  BusOutput=off  SignalInfo={ 'Gyro_z', '0', '16', 'LE', 'unsigned', 'Standard', '0', '1', '0', '-Inf', 'Inf'; 'Gyro_y', '16', '16', 'LE', 'unsigned', 'Standard', '0', '1', '0', '-Inf', 'Inf'; 'Gyro_x', '32', '16', 'LE', 'unsigned', 'Standard', '0', '1', '0', '-Inf', 'Inf' }
      settings: SourceProductName=Vehicle Network Toolbox  SourceProductBaseCode=VN  DataFormat=manually specified signals
  CAN Pack2 : canmsglib/CAN Pack  MsgList=(none)  MsgName=Motor Heartbeat FL  MsgIDType=Standard (11-bit identifier)  MsgIdentifier=113  MsgLength=5  Remote=off  ApplyMinMax=off  BusOutput=off  SignalInfo={ 'MotorT', '0', '12', 'LE', 'unsigned', 'Standard', '0', '1', '0', '-Inf', 'Inf'; 'GearboxT', '16', '12', 'LE', 'unsigned', 'Standard', '0', '1', '0', '-Inf', 'Inf'; 'Suspension', '28', '12', 'LE', 'unsigned', 'Standard', '0', '1', '0', '-Inf', 'Inf' }
      settings: SourceProductName=Vehicle Network Toolbox  SourceProductBaseCode=VN  DataFormat=manually specified signals
  CAN Pack3 : canmsglib/CAN Pack  MsgList=(none)  MsgName=Error GearboxT FL  MsgIDType=Standard (11-bit identifier)  MsgIdentifier=133  MsgLength=1  Remote=off  ApplyMinMax=off  BusOutput=off  SignalInfo={ 'Signal1', '0', '1', 'LE', 'unsigned', 'Standard', '0', '1', '0', '-Inf', 'Inf' }
      settings: SourceProductName=Vehicle Network Toolbox  SourceProductBaseCode=VN  DataFormat=manually specified signals
  CAN Pack4 : canmsglib/CAN Pack  MsgList=(none)  MsgName=Error MotorT FL  MsgIDType=Standard (11-bit identifier)  MsgIdentifier=123  MsgLength=1  Remote=off  ApplyMinMax=off  BusOutput=off  SignalInfo={ 'Signal1', '0', '1', 'LE', 'unsigned', 'Standard', '0', '1', '0', '-Inf', 'Inf' }
      settings: SourceProductName=Vehicle Network Toolbox  SourceProductBaseCode=VN  DataFormat=manually specified signals
  CAN Transmit : canlib/CAN Transmit  BlockHandle=331.0002  Device=MathWorks Virtual 1 (Channel 1)  DeviceMenu=MathWorks Virtual 1 (Channel 1)  ObjConstructor=canChannel('MathWorks', 'Virtual 1', 1)  EnablePeriodicTransmit=on  MessagePeriod=0.250
      settings: SourceProductName=Vehicle Network Toolbox  SourceProductBaseCode=VN
  CAN Transmit1 : canlib/CAN Transmit  BlockHandle=332.0002  Device=MathWorks Virtual 1 (Channel 1)  DeviceMenu=MathWorks Virtual 1 (Channel 1)  ObjConstructor=canChannel('MathWorks', 'Virtual 1', 1)  EnablePeriodicTransmit=on  MessagePeriod=0.250
      settings: SourceProductName=Vehicle Network Toolbox  SourceProductBaseCode=VN
  CAN Transmit2 : canlib/CAN Transmit  BlockHandle=333.0002  Device=MathWorks Virtual 1 (Channel 1)  DeviceMenu=MathWorks Virtual 1 (Channel 1)  ObjConstructor=canChannel('MathWorks', 'Virtual 1', 1)  EnablePeriodicTransmit=on  MessagePeriod=0.250
      settings: SourceProductName=Vehicle Network Toolbox  SourceProductBaseCode=VN
  CAN Transmit3 : canlib/CAN Transmit  BlockHandle=334.0002  Device=MathWorks Virtual 1 (Channel 1)  DeviceMenu=MathWorks Virtual 1 (Channel 1)  ObjConstructor=canChannel('MathWorks', 'Virtual 1', 1)  EnablePeriodicTransmit=on  MessagePeriod=0.250
      settings: SourceProductName=Vehicle Network Toolbox  SourceProductBaseCode=VN
  CAN Transmit4 : canlib/CAN Transmit  BlockHandle=335.0002  Device=MathWorks Virtual 1 (Channel 1)  DeviceMenu=MathWorks Virtual 1 (Channel 1)  ObjConstructor=canChannel('MathWorks', 'Virtual 1', 1)  EnablePeriodicTransmit=on  MessagePeriod=0.250
      settings: SourceProductName=Vehicle Network Toolbox  SourceProductBaseCode=VN
  Data Type Conversion5 : DataTypeConversion  OutDataTypeStr=uint8
  Data Type Conversion6 : DataTypeConversion  OutDataTypeStr=uint8
  Error1 : Switch  Criteria=u2 > Threshold  Threshold=1000
  Error2 : Switch  Criteria=u2 > Threshold  Threshold=1000
  Out3 : Outport
  Out4 : Outport  Port=2
  wires:
  0/1 -> Error1/3
  CAN Pack4/1 -> CAN Transmit4/1
  Data Type Conversion6/1 -> CAN Pack4/1
  In3/1 -> CAN Pack/3
  Error1/1 -> Out3/1, Data Type Conversion5/1
  In6/1 -> CAN Pack1/3
  Data Type Conversion5/1 -> CAN Pack3/1
  In8/1 -> Error1/2, CAN Pack2/2
  3/1 -> Error2/1
  2/1 -> Error2/3
  In9/1 -> Error2/2, CAN Pack2/1
  1/1 -> Error1/1
  Error2/1 -> Out4/1, Data Type Conversion6/1
  CAN Pack2/1 -> CAN Transmit2/1
  CAN Pack3/1 -> CAN Transmit3/1
  CAN Pack/1 -> CAN Transmit/1
  CAN Pack1/1 -> CAN Transmit1/1
  In2/1 -> CAN Pack/2
  In4/1 -> CAN Pack1/1
  In5/1 -> CAN Pack1/2
  In1/1 -> CAN Pack/1
  In7/1 -> CAN Pack2/3

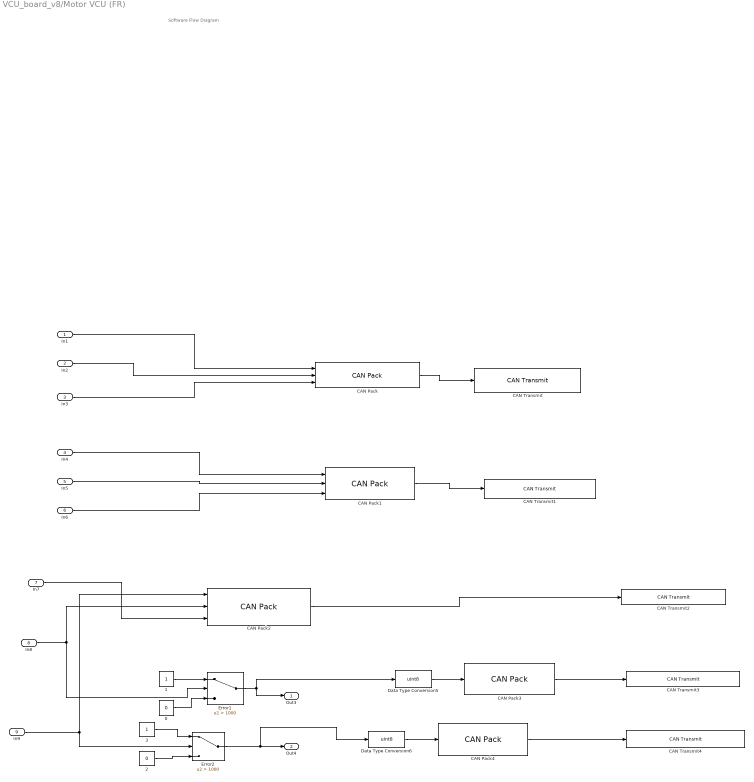
== system VCU_board_v8/Motor VCU (FR) ==
  note: Software Flow Diagram
  In1 : Inport
  In2 : Inport  Port=2
  In3 : Inport  Port=3
  In4 : Inport  Port=4
  In5 : Inport  Port=5
  In6 : Inport  Port=6
  In7 : Inport  Port=7
  In8 : Inport  Port=8
  In9 : Inport  Port=9
  0 : Constant  Value=0
  1 : Constant
  2 : Constant  Value=0
  3 : Constant
  CAN Pack : canmsglib/CAN Pack  MsgList=(none)  MsgName=Accel  MsgIDType=Standard (11-bit identifier)  MsgIdentifier=151  MsgLength=6  Remote=off  ApplyMinMax=off  BusOutput=off  SignalInfo={ 'Accel_z', '0', '16', 'LE', 'unsigned', 'Standard', '0', '1', '0', '-Inf', 'Inf'; 'Accel_y', '16', '16', 'LE', 'unsigned', 'Standard', '0', '1', '0', '-Inf', 'Inf'; 'Accel_x', '32', '16', 'LE', 'unsigned', 'Standard', '0', '1', '0', '-Inf', 'Inf' }
      settings: SourceProductName=Vehicle Network Toolbox  SourceProductBaseCode=VN  DataFormat=manually specified signals
  CAN Pack1 : canmsglib/CAN Pack  MsgList=(none)  MsgName=CAN Msg  MsgIDType=Standard (11-bit identifier)  MsgIdentifier=141  MsgLength=6  Remote=off  ApplyMinMax=off  BusOutput=off  SignalInfo={ 'Gyro_z', '0', '16', 'LE', 'unsigned', 'Standard', '0', '1', '0', '-Inf', 'Inf'; 'Gyro_y', '16', '16', 'LE', 'unsigned', 'Standard', '0', '1', '0', '-Inf', 'Inf'; 'Gyro_x', '32', '16', 'LE', 'unsigned', 'Standard', '0', '1', '0', '-Inf', 'Inf' }
      settings: SourceProductName=Vehicle Network Toolbox  SourceProductBaseCode=VN  DataFormat=manually specified signals
  CAN Pack2 : canmsglib/CAN Pack  MsgList=(none)  MsgName=Motor Heartbeat  MsgIDType=Standard (11-bit identifier)  MsgIdentifier=111  MsgLength=5  Remote=off  ApplyMinMax=off  BusOutput=off  SignalInfo={ 'MotorT', '0', '12', 'LE', 'unsigned', 'Standard', '0', '1', '0', '-Inf', 'Inf'; 'GearboxT', '16', '12', 'LE', 'unsigned', 'Standard', '0', '1', '0', '-Inf', 'Inf'; 'Suspension', '28', '12', 'LE', 'unsigned', 'Standard', '0', '1', '0', '-Inf', 'Inf' }
      settings: SourceProductName=Vehicle Network Toolbox  SourceProductBaseCode=VN  DataFormat=manually specified signals
  CAN Pack3 : canmsglib/CAN Pack  MsgList=(none)  MsgName=CAN Msg  MsgIDType=Standard (11-bit identifier)  MsgIdentifier=131  MsgLength=1  Remote=off  ApplyMinMax=off  BusOutput=off  SignalInfo={ 'Signal1', '0', '1', 'LE', 'unsigned', 'Standard', '0', '1', '0', '-Inf', 'Inf' }
      settings: SourceProductName=Vehicle Network Toolbox  SourceProductBaseCode=VN  DataFormat=manually specified signals
  CAN Pack4 : canmsglib/CAN Pack  MsgList=(none)  MsgName=CAN Msg  MsgIDType=Standard (11-bit identifier)  MsgIdentifier=121  MsgLength=1  Remote=off  ApplyMinMax=off  BusOutput=off  SignalInfo={ 'Signal1', '0', '1', 'LE', 'unsigned', 'Standard', '0', '1', '0', '-Inf', 'Inf' }
      settings: SourceProductName=Vehicle Network Toolbox  SourceProductBaseCode=VN  DataFormat=manually specified signals
  CAN Transmit : canlib/CAN Transmit  BlockHandle=331.0002  Device=MathWorks Virtual 1 (Channel 1)  DeviceMenu=MathWorks Virtual 1 (Channel 1)  ObjConstructor=canChannel('MathWorks', 'Virtual 1', 1)  EnablePeriodicTransmit=on  MessagePeriod=0.250
      settings: SourceProductName=Vehicle Network Toolbox  SourceProductBaseCode=VN
  CAN Transmit1 : canlib/CAN Transmit  BlockHandle=332.0002  Device=MathWorks Virtual 1 (Channel 1)  DeviceMenu=MathWorks Virtual 1 (Channel 1)  ObjConstructor=canChannel('MathWorks', 'Virtual 1', 1)  EnablePeriodicTransmit=on  MessagePeriod=0.250
      settings: SourceProductName=Vehicle Network Toolbox  SourceProductBaseCode=VN
  CAN Transmit2 : canlib/CAN Transmit  BlockHandle=333.0002  Device=MathWorks Virtual 1 (Channel 1)  DeviceMenu=MathWorks Virtual 1 (Channel 1)  ObjConstructor=canChannel('MathWorks', 'Virtual 1', 1)  EnablePeriodicTransmit=on  MessagePeriod=0.250
      settings: SourceProductName=Vehicle Network Toolbox  SourceProductBaseCode=VN
  CAN Transmit3 : canlib/CAN Transmit  BlockHandle=334.0002  Device=MathWorks Virtual 1 (Channel 1)  DeviceMenu=MathWorks Virtual 1 (Channel 1)  ObjConstructor=canChannel('MathWorks', 'Virtual 1', 1)  EnablePeriodicTransmit=on  MessagePeriod=0.250
      settings: SourceProductName=Vehicle Network Toolbox  SourceProductBaseCode=VN
  CAN Transmit4 : canlib/CAN Transmit  BlockHandle=335.0002  Device=MathWorks Virtual 1 (Channel 1)  DeviceMenu=MathWorks Virtual 1 (Channel 1)  ObjConstructor=canChannel('MathWorks', 'Virtual 1', 1)  EnablePeriodicTransmit=on  MessagePeriod=0.250
      settings: SourceProductName=Vehicle Network Toolbox  SourceProductBaseCode=VN
  Data Type Conversion5 : DataTypeConversion  OutDataTypeStr=uint8
  Data Type Conversion6 : DataTypeConversion  OutDataTypeStr=uint8
  Error1 : Switch  Criteria=u2 > Threshold  Threshold=1000
  Error2 : Switch  Criteria=u2 > Threshold  Threshold=1000
  Out3 : Outport
  Out4 : Outport  Port=2
  wires:
  0/1 -> Error1/3
  CAN Pack4/1 -> CAN Transmit4/1
  Data Type Conversion6/1 -> CAN Pack4/1
  In3/1 -> CAN Pack/3
  Error1/1 -> Out3/1, Data Type Conversion5/1
  In6/1 -> CAN Pack1/3
  Data Type Conversion5/1 -> CAN Pack3/1
  In8/1 -> Error1/2, CAN Pack2/2
  3/1 -> Error2/1
  2/1 -> Error2/3
  In9/1 -> Error2/2, CAN Pack2/1
  1/1 -> Error1/1
  Error2/1 -> Out4/1, Data Type Conversion6/1
  CAN Pack2/1 -> CAN Transmit2/1
  CAN Pack3/1 -> CAN Transmit3/1
  CAN Pack/1 -> CAN Transmit/1
  CAN Pack1/1 -> CAN Transmit1/1
  In2/1 -> CAN Pack/2
  In4/1 -> CAN Pack1/1
  In5/1 -> CAN Pack1/2
  In1/1 -> CAN Pack/1
  In7/1 -> CAN Pack2/3

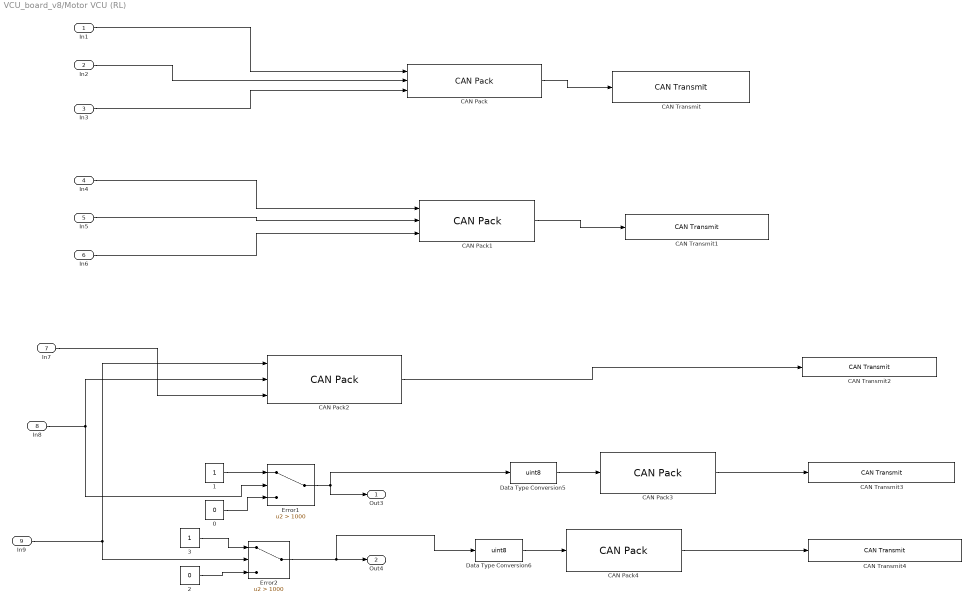
== system VCU_board_v8/Motor VCU (RL) ==
  In1 : Inport
  In2 : Inport  Port=2
  In3 : Inport  Port=3
  In4 : Inport  Port=4
  In5 : Inport  Port=5
  In6 : Inport  Port=6
  In7 : Inport  Port=7
  In8 : Inport  Port=8
  In9 : Inport  Port=9
  0 : Constant  Value=0
  1 : Constant
  2 : Constant  Value=0
  3 : Constant
  CAN Pack : canmsglib/CAN Pack  MsgList=(none)  MsgName=Accel RR  MsgIDType=Standard (11-bit identifier)  MsgIdentifier=154  MsgLength=6  Remote=off  ApplyMinMax=off  BusOutput=off  SignalInfo={ 'Accel_z', '0', '16', 'LE', 'unsigned', 'Standard', '0', '1', '0', '-Inf', 'Inf'; 'Accel_y', '16', '16', 'LE', 'unsigned', 'Standard', '0', '1', '0', '-Inf', 'Inf'; 'Accel_x', '32', '16', 'LE', 'unsigned', 'Standard', '0', '1', '0', '-Inf', 'Inf' }
      settings: SourceProductName=Vehicle Network Toolbox  SourceProductBaseCode=VN  DataFormat=manually specified signals
  CAN Pack1 : canmsglib/CAN Pack  MsgList=(none)  MsgName=Gyro RL  MsgIDType=Standard (11-bit identifier)  MsgIdentifier=144  MsgLength=6  Remote=off  ApplyMinMax=off  BusOutput=off  SignalInfo={ 'Gyro_z', '0', '16', 'LE', 'unsigned', 'Standard', '0', '1', '0', '-Inf', 'Inf'; 'Gyro_y', '16', '16', 'LE', 'unsigned', 'Standard', '0', '1', '0', '-Inf', 'Inf'; 'Gyro_x', '32', '16', 'LE', 'unsigned', 'Standard', '0', '1', '0', '-Inf', 'Inf' }
      settings: SourceProductName=Vehicle Network Toolbox  SourceProductBaseCode=VN  DataFormat=manually specified signals
  CAN Pack2 : canmsglib/CAN Pack  MsgList=(none)  MsgName=Motor Heartbeat RL  MsgIDType=Standard (11-bit identifier)  MsgIdentifier=114  MsgLength=5  Remote=off  ApplyMinMax=off  BusOutput=off  SignalInfo={ 'MotorT', '0', '12', 'LE', 'unsigned', 'Standard', '0', '1', '0', '-Inf', 'Inf'; 'GearboxT', '16', '12', 'LE', 'unsigned', 'Standard', '0', '1', '0', '-Inf', 'Inf'; 'Suspension', '28', '12', 'LE', 'unsigned', 'Standard', '0', '1', '0', '-Inf', 'Inf' }
      settings: SourceProductName=Vehicle Network Toolbox  SourceProductBaseCode=VN  DataFormat=manually specified signals
  CAN Pack3 : canmsglib/CAN Pack  MsgList=(none)  MsgName=Error GearboxT RL  MsgIDType=Standard (11-bit identifier)  MsgIdentifier=134  MsgLength=1  Remote=off  ApplyMinMax=off  BusOutput=off  SignalInfo={ 'Signal1', '0', '1', 'LE', 'unsigned', 'Standard', '0', '1', '0', '-Inf', 'Inf' }
      settings: SourceProductName=Vehicle Network Toolbox  SourceProductBaseCode=VN  DataFormat=manually specified signals
  CAN Pack4 : canmsglib/CAN Pack  MsgList=(none)  MsgName=Error MotorT RL  MsgIDType=Standard (11-bit identifier)  MsgIdentifier=124  MsgLength=1  Remote=off  ApplyMinMax=off  BusOutput=off  SignalInfo={ 'Signal1', '0', '1', 'LE', 'unsigned', 'Standard', '0', '1', '0', '-Inf', 'Inf' }
      settings: SourceProductName=Vehicle Network Toolbox  SourceProductBaseCode=VN  DataFormat=manually specified signals
  CAN Transmit : canlib/CAN Transmit  BlockHandle=331.0002  Device=MathWorks Virtual 1 (Channel 1)  DeviceMenu=MathWorks Virtual 1 (Channel 1)  ObjConstructor=canChannel('MathWorks', 'Virtual 1', 1)  EnablePeriodicTransmit=on  MessagePeriod=0.250
      settings: SourceProductName=Vehicle Network Toolbox  SourceProductBaseCode=VN
  CAN Transmit1 : canlib/CAN Transmit  BlockHandle=332.0002  Device=MathWorks Virtual 1 (Channel 1)  DeviceMenu=MathWorks Virtual 1 (Channel 1)  ObjConstructor=canChannel('MathWorks', 'Virtual 1', 1)  EnablePeriodicTransmit=on  MessagePeriod=0.250
      settings: SourceProductName=Vehicle Network Toolbox  SourceProductBaseCode=VN
  CAN Transmit2 : canlib/CAN Transmit  BlockHandle=333.0002  Device=MathWorks Virtual 1 (Channel 1)  DeviceMenu=MathWorks Virtual 1 (Channel 1)  ObjConstructor=canChannel('MathWorks', 'Virtual 1', 1)  EnablePeriodicTransmit=on  MessagePeriod=0.250
      settings: SourceProductName=Vehicle Network Toolbox  SourceProductBaseCode=VN
  CAN Transmit3 : canlib/CAN Transmit  BlockHandle=334.0002  Device=MathWorks Virtual 1 (Channel 1)  DeviceMenu=MathWorks Virtual 1 (Channel 1)  ObjConstructor=canChannel('MathWorks', 'Virtual 1', 1)  EnablePeriodicTransmit=on  MessagePeriod=0.250
      settings: SourceProductName=Vehicle Network Toolbox  SourceProductBaseCode=VN
  CAN Transmit4 : canlib/CAN Transmit  BlockHandle=335.0002  Device=MathWorks Virtual 1 (Channel 1)  DeviceMenu=MathWorks Virtual 1 (Channel 1)  ObjConstructor=canChannel('MathWorks', 'Virtual 1', 1)  EnablePeriodicTransmit=on  MessagePeriod=0.250
      settings: SourceProductName=Vehicle Network Toolbox  SourceProductBaseCode=VN
  Data Type Conversion5 : DataTypeConversion  OutDataTypeStr=uint8
  Data Type Conversion6 : DataTypeConversion  OutDataTypeStr=uint8
  Error1 : Switch  Criteria=u2 > Threshold  Threshold=1000
  Error2 : Switch  Criteria=u2 > Threshold  Threshold=1000
  Out3 : Outport
  Out4 : Outport  Port=2
  wires:
  0/1 -> Error1/3
  CAN Pack4/1 -> CAN Transmit4/1
  Data Type Conversion6/1 -> CAN Pack4/1
  In3/1 -> CAN Pack/3
  Error1/1 -> Out3/1, Data Type Conversion5/1
  In6/1 -> CAN Pack1/3
  Data Type Conversion5/1 -> CAN Pack3/1
  In8/1 -> Error1/2, CAN Pack2/2
  3/1 -> Error2/1
  2/1 -> Error2/3
  In9/1 -> Error2/2, CAN Pack2/1
  1/1 -> Error1/1
  Error2/1 -> Out4/1, Data Type Conversion6/1
  CAN Pack2/1 -> CAN Transmit2/1
  CAN Pack3/1 -> CAN Transmit3/1
  CAN Pack/1 -> CAN Transmit/1
  CAN Pack1/1 -> CAN Transmit1/1
  In2/1 -> CAN Pack/2
  In4/1 -> CAN Pack1/1
  In5/1 -> CAN Pack1/2
  In1/1 -> CAN Pack/1
  In7/1 -> CAN Pack2/3

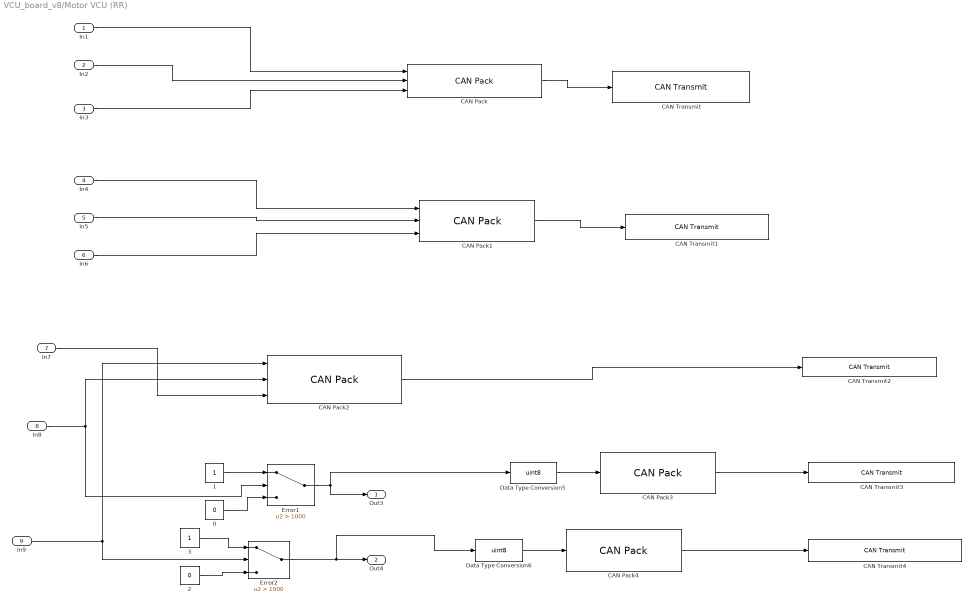
== system VCU_board_v8/Motor VCU (RR) ==
  In1 : Inport
  In2 : Inport  Port=2
  In3 : Inport  Port=3
  In4 : Inport  Port=4
  In5 : Inport  Port=5
  In6 : Inport  Port=6
  In7 : Inport  Port=7
  In8 : Inport  Port=8
  In9 : Inport  Port=9
  0 : Constant  Value=0
  1 : Constant
  2 : Constant  Value=0
  3 : Constant
  CAN Pack : canmsglib/CAN Pack  MsgList=(none)  MsgName=Accel RR  MsgIDType=Standard (11-bit identifier)  MsgIdentifier=152  MsgLength=6  Remote=off  ApplyMinMax=off  BusOutput=off  SignalInfo={ 'Accel_z', '0', '16', 'LE', 'unsigned', 'Standard', '0', '1', '0', '-Inf', 'Inf'; 'Accel_y', '16', '16', 'LE', 'unsigned', 'Standard', '0', '1', '0', '-Inf', 'Inf'; 'Accel_x', '32', '16', 'LE', 'unsigned', 'Standard', '0', '1', '0', '-Inf', 'Inf' }
      settings: SourceProductName=Vehicle Network Toolbox  SourceProductBaseCode=VN  DataFormat=manually specified signals
  CAN Pack1 : canmsglib/CAN Pack  MsgList=(none)  MsgName=Gyro RR  MsgIDType=Standard (11-bit identifier)  MsgIdentifier=142  MsgLength=6  Remote=off  ApplyMinMax=off  BusOutput=off  SignalInfo={ 'Gyro_z', '0', '16', 'LE', 'unsigned', 'Standard', '0', '1', '0', '-Inf', 'Inf'; 'Gyro_y', '16', '16', 'LE', 'unsigned', 'Standard', '0', '1', '0', '-Inf', 'Inf'; 'Gyro_x', '32', '16', 'LE', 'unsigned', 'Standard', '0', '1', '0', '-Inf', 'Inf' }
      settings: SourceProductName=Vehicle Network Toolbox  SourceProductBaseCode=VN  DataFormat=manually specified signals
  CAN Pack2 : canmsglib/CAN Pack  MsgList=(none)  MsgName=Motor Heartbeat RR  MsgIDType=Standard (11-bit identifier)  MsgIdentifier=112  MsgLength=5  Remote=off  ApplyMinMax=off  BusOutput=off  SignalInfo={ 'MotorT', '0', '12', 'LE', 'unsigned', 'Standard', '0', '1', '0', '-Inf', 'Inf'; 'GearboxT', '16', '12', 'LE', 'unsigned', 'Standard', '0', '1', '0', '-Inf', 'Inf'; 'Suspension', '28', '12', 'LE', 'unsigned', 'Standard', '0', '1', '0', '-Inf', 'Inf' }
      settings: SourceProductName=Vehicle Network Toolbox  SourceProductBaseCode=VN  DataFormat=manually specified signals
  CAN Pack3 : canmsglib/CAN Pack  MsgList=(none)  MsgName=Error GearboxT RR  MsgIDType=Standard (11-bit identifier)  MsgIdentifier=132  MsgLength=1  Remote=off  ApplyMinMax=off  BusOutput=off  SignalInfo={ 'Signal1', '0', '1', 'LE', 'unsigned', 'Standard', '0', '1', '0', '-Inf', 'Inf' }
      settings: SourceProductName=Vehicle Network Toolbox  SourceProductBaseCode=VN  DataFormat=manually specified signals
  CAN Pack4 : canmsglib/CAN Pack  MsgList=(none)  MsgName=Error MotorT RR  MsgIDType=Standard (11-bit identifier)  MsgIdentifier=122  MsgLength=1  Remote=off  ApplyMinMax=off  BusOutput=off  SignalInfo={ 'Signal1', '0', '1', 'LE', 'unsigned', 'Standard', '0', '1', '0', '-Inf', 'Inf' }
      settings: SourceProductName=Vehicle Network Toolbox  SourceProductBaseCode=VN  DataFormat=manually specified signals
  CAN Transmit : canlib/CAN Transmit  BlockHandle=331.0002  Device=MathWorks Virtual 1 (Channel 1)  DeviceMenu=MathWorks Virtual 1 (Channel 1)  ObjConstructor=canChannel('MathWorks', 'Virtual 1', 1)  EnablePeriodicTransmit=on  MessagePeriod=0.250
      settings: SourceProductName=Vehicle Network Toolbox  SourceProductBaseCode=VN
  CAN Transmit1 : canlib/CAN Transmit  BlockHandle=332.0002  Device=MathWorks Virtual 1 (Channel 1)  DeviceMenu=MathWorks Virtual 1 (Channel 1)  ObjConstructor=canChannel('MathWorks', 'Virtual 1', 1)  EnablePeriodicTransmit=on  MessagePeriod=0.250
      settings: SourceProductName=Vehicle Network Toolbox  SourceProductBaseCode=VN
  CAN Transmit2 : canlib/CAN Transmit  BlockHandle=333.0002  Device=MathWorks Virtual 1 (Channel 1)  DeviceMenu=MathWorks Virtual 1 (Channel 1)  ObjConstructor=canChannel('MathWorks', 'Virtual 1', 1)  EnablePeriodicTransmit=on  MessagePeriod=0.250
      settings: SourceProductName=Vehicle Network Toolbox  SourceProductBaseCode=VN
  CAN Transmit3 : canlib/CAN Transmit  BlockHandle=334.0002  Device=MathWorks Virtual 1 (Channel 1)  DeviceMenu=MathWorks Virtual 1 (Channel 1)  ObjConstructor=canChannel('MathWorks', 'Virtual 1', 1)  EnablePeriodicTransmit=on  MessagePeriod=0.250
      settings: SourceProductName=Vehicle Network Toolbox  SourceProductBaseCode=VN
  CAN Transmit4 : canlib/CAN Transmit  BlockHandle=335.0002  Device=MathWorks Virtual 1 (Channel 1)  DeviceMenu=MathWorks Virtual 1 (Channel 1)  ObjConstructor=canChannel('MathWorks', 'Virtual 1', 1)  EnablePeriodicTransmit=on  MessagePeriod=0.250
      settings: SourceProductName=Vehicle Network Toolbox  SourceProductBaseCode=VN
  Data Type Conversion5 : DataTypeConversion  OutDataTypeStr=uint8
  Data Type Conversion6 : DataTypeConversion  OutDataTypeStr=uint8
  Error1 : Switch  Criteria=u2 > Threshold  Threshold=1000
  Error2 : Switch  Criteria=u2 > Threshold  Threshold=1000
  Out3 : Outport
  Out4 : Outport  Port=2
  wires:
  0/1 -> Error1/3
  CAN Pack4/1 -> CAN Transmit4/1
  Data Type Conversion6/1 -> CAN Pack4/1
  In3/1 -> CAN Pack/3
  Error1/1 -> Out3/1, Data Type Conversion5/1
  In6/1 -> CAN Pack1/3
  Data Type Conversion5/1 -> CAN Pack3/1
  In8/1 -> Error1/2, CAN Pack2/2
  3/1 -> Error2/1
  2/1 -> Error2/3
  In9/1 -> Error2/2, CAN Pack2/1
  1/1 -> Error1/1
  Error2/1 -> Out4/1, Data Type Conversion6/1
  CAN Pack2/1 -> CAN Transmit2/1
  CAN Pack3/1 -> CAN Transmit3/1
  CAN Pack/1 -> CAN Transmit/1
  CAN Pack1/1 -> CAN Transmit1/1
  In2/1 -> CAN Pack/2
  In4/1 -> CAN Pack1/1
  In5/1 -> CAN Pack1/2
  In1/1 -> CAN Pack/1
  In7/1 -> CAN Pack2/3
